simulink model "Despejes_TF"  (R2014a)
settings: Solver=ode45  StartTime=0.0  StopTime=10.0  RelTol=1e-3
values from neighbouring files (symbols this model uses):
  b = 1.1    [TP1.m]
  J = 15    [TP1.m]
  K = 6.7628    [TP1.m]
  L = 2.886e-3    (= 0.002886)    [TP1.m]    (also in retrato3d.m = W\A*W)
  R = 50.296e-3    (= 0.050296)    [TP1.m]
  s = tf([1,0],1)    [TP1.m]
undefined symbols (not defined in the file or in its folder): Js, Ls
settings Model: Creator=lraff  LastModifiedBy=lraff

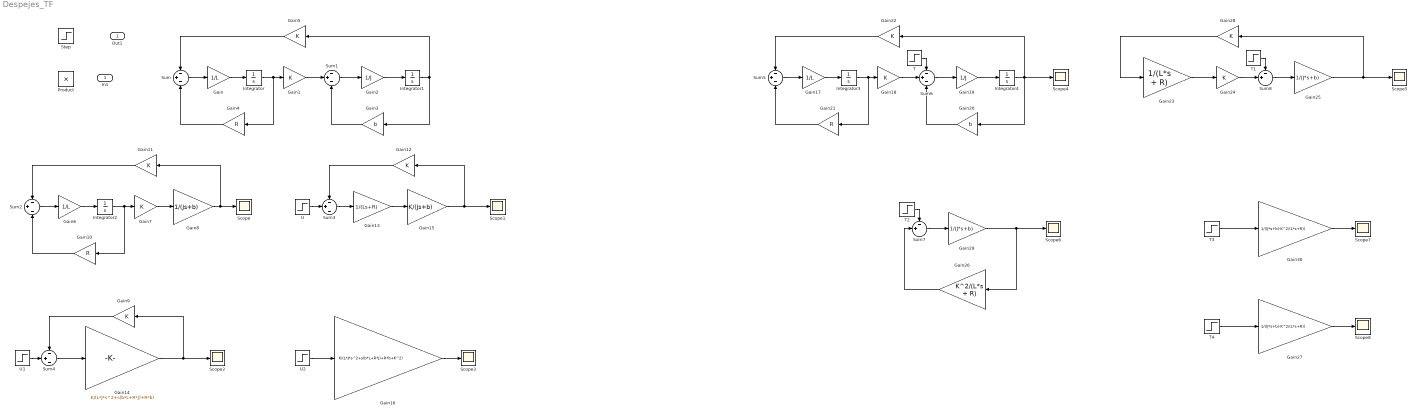
== system Despejes_TF ==
  In1 : Inport
  Gain : Gain  Gain=1/L
  Gain{1,5,7,9,11..12,18,22,24,28} (10 alike) : Gain  Gain=K
  Gain10 : Gain  Gain=R
  Gain13 : Gain  Gain=1/(Ls+R)
  Gain14 : Gain  Gain=K/(L*J*s^2+s(b*L+R*J)+R*b)
  Gain15 : Gain  Gain=K/(Js+b)
  Gain16 : Gain  Gain=K/(L*J*s^2+s(b*L+R*J)+R*b+K^2)
  Gain17 : Gain  Gain=1/L
  Gain19 : Gain  Gain=1/J
  Gain2 : Gain  Gain=1/J
  Gain20 : Gain  Gain=b
  Gain21 : Gain  Gain=R
  Gain23 : Gain  Gain=1/(L*s + R)
  Gain25 : Gain  Gain=1/(J*s+b)
  Gain26 : Gain  Gain=K^2/(L*s + R)
  Gain27 : Gain  Gain=1/((J*s+b)-K^2/(L*s+R))
  Gain29 : Gain  Gain=1/(J*s+b)
  Gain3 : Gain  Gain=b
  Gain30 : Gain  Gain=1/((J*s+b)-K^2/(L*s+R))
  Gain4 : Gain  Gain=R
  Gain6 : Gain  Gain=1/L
  Gain8 : Gain  Gain=1/(Js+b)
  Integrator{,1..4} (5 alike) : Integrator
  Product : Product
  Scope{,1..8} (9 alike) : Scope
      Scope2 settings: SaveName=ScopeData2
      Scope3 settings: SaveName=ScopeData3
      Scope4 settings: SaveName=ScopeData4
      Scope5 settings: SaveName=ScopeData5
      Scope6 settings: SaveName=ScopeData6
      Scope7 settings: SaveName=ScopeData7
      Scope8 settings: SaveName=ScopeData8
  Step : Step  SampleTime=0
  Sum{,1..6} (7 alike) : Sum  Inputs=-+-
  Sum7 : Sum  Inputs=-+|
  Sum8 : Sum  Inputs=-+|
  T{,1..4} (5 alike) : Step  SampleTime=0
  U : Step  SampleTime=0
  U1 : Step  SampleTime=0
  U2 : Step  SampleTime=0
  Out1 : Outport
  wires:
  Sum/1 -> Gain/1
  Gain/1 -> Integrator/1
  Integrator/1 -> Gain4/1, Gain1/1
  Gain1/1 -> Sum1/2
  Sum1/1 -> Gain2/1
  Gain2/1 -> Integrator1/1
  Integrator1/1 -> Gain5/1, Gain3/1
  Gain3/1 -> Sum1/3
  Gain4/1 -> Sum/3
  Gain5/1 -> Sum/1
  Sum2/1 -> Gain6/1
  Gain6/1 -> Integrator2/1
  Integrator2/1 -> Gain10/1, Gain7/1
  Gain7/1 -> Gain8/1
  Gain8/1 -> Scope/1, Gain11/1
  Gain10/1 -> Sum2/3
  Gain11/1 -> Sum2/1
  Sum3/1 -> Gain13/1
  Gain13/1 -> Gain15/1
  Gain15/1 -> Scope1/1, Gain12/1
  Gain12/1 -> Sum3/1
  U/1 -> Sum3/2
  Sum4/1 -> Gain14/1
  Gain14/1 -> Scope2/1, Gain9/1
  Gain9/1 -> Sum4/1
  U1/1 -> Sum4/2
  U2/1 -> Gain16/1
  Gain16/1 -> Scope3/1
  Sum5/1 -> Gain17/1
  Gain17/1 -> Integrator3/1
  Integrator3/1 -> Gain21/1, Gain18/1
  Gain18/1 -> Sum6/2
  Sum6/1 -> Gain19/1
  Gain19/1 -> Integrator4/1
  Gain20/1 -> Sum6/3
  Gain21/1 -> Sum5/3
  Gain22/1 -> Sum5/1
  T/1 -> Sum6/1
  Integrator4/1 -> Scope4/1, Gain22/1, Gain20/1
  Gain28/1 -> Gain23/1
  Gain23/1 -> Gain24/1
  Gain24/1 -> Sum8/2
  Sum8/1 -> Gain25/1
  T1/1 -> Sum8/1
  Gain25/1 -> Scope5/1, Gain28/1
  Gain29/1 -> Gain26/1, Scope6/1
  Gain26/1 -> Sum7/2
  Sum7/1 -> Gain29/1
  T2/1 -> Sum7/1
  Gain30/1 -> Scope7/1
  T3/1 -> Gain30/1
  Gain27/1 -> Scope8/1
  T4/1 -> Gain27/1
